simulink model "gm_parallel_8_delay_compensation"  (R2022a)
settings: Solver=FixedStepDiscrete  StartTime=0.0  StopTime=10.0  RelTol=1e-3
undefined symbols (not defined in the file or in its folder): f_c, L_d, L_q, L_x, L_y, p, psi_pm, R_ph
libraries: hdlmdlgenlib x30
settings Model: Creator=Andre Merx  LastModifiedBy=Andre Merx
settings SolverCC: AlgebraicLoopSolver=TrustRegion
settings DataIOCC: LimitDataPoints=on  SaveOutput=off  SaveTime=off
settings OptimizationCC: BlockReduction=off  ConditionallyExecuteInputs=off  DefaultParameterBehavior=Inlined  LifeSpan=inf
settings DebuggingCC: AlgebraicLoopMsg=error  InheritedTsInSrcMsg=none  SingleTaskRateTransMsg=error  UnconnectedInputMsg=warning  UnconnectedOutputMsg=warning  UnconnectedLineMsg=warning  AllowSymbolicDim=off  StrictBusMsg=ErrorOnBusTreatedAsVector  SFUnexpectedBacktrackingDiag=warning  SFNoUnconditionalDefaultTransitionDiag=warning  SFExecutionAtInitializationDiag=none  SFMachineParentedDataDiag=warning  ArithmeticOperatorsInVariantConditions=warning
settings HardwareCC: ProdBitPerPointer=32  ProdBitPerSizeT=32  ProdBitPerPtrDiffT=32  ProdLargestAtomicFloat=None  ProdIntDivRoundTo=Undefined  ProdEndianess=Unspecified  ProdWordSize=32  ProdHWDeviceType=ASIC/FPGA->ASIC/FPGA  ProdEqTarget=off
settings SFSimCC: SimUseLocalCustomCode=off  CustomCodeUndefinedFunction=UseInterfaceOnly
settings RTWCC: RTWUseLocalCustomCode=off
settings CodeAppCC: StateflowObjectComments=on
settings GRTTargetCC: TargetLangStandard=C89/C90 (ANSI)
settings ConfigComp: CovScope=ReferencedModels  CovMetricSettings=dw  CovSaveCumulativeToWorkspaceVar=on  CovSaveSingleToWorkspaceVar=on  CovExternalEMLEnable=off  CovSFcnEnable=off

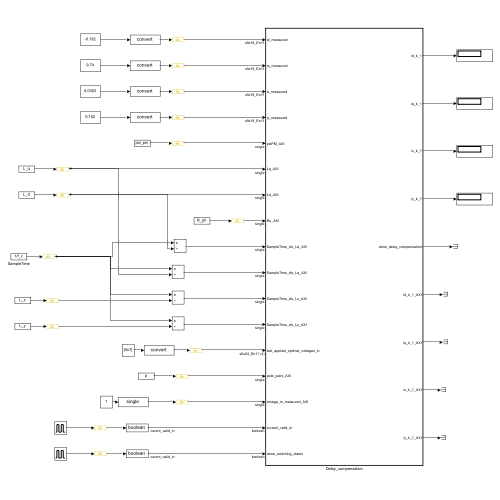
[thumbnail: Simulink's stored preview of the top-level diagram]
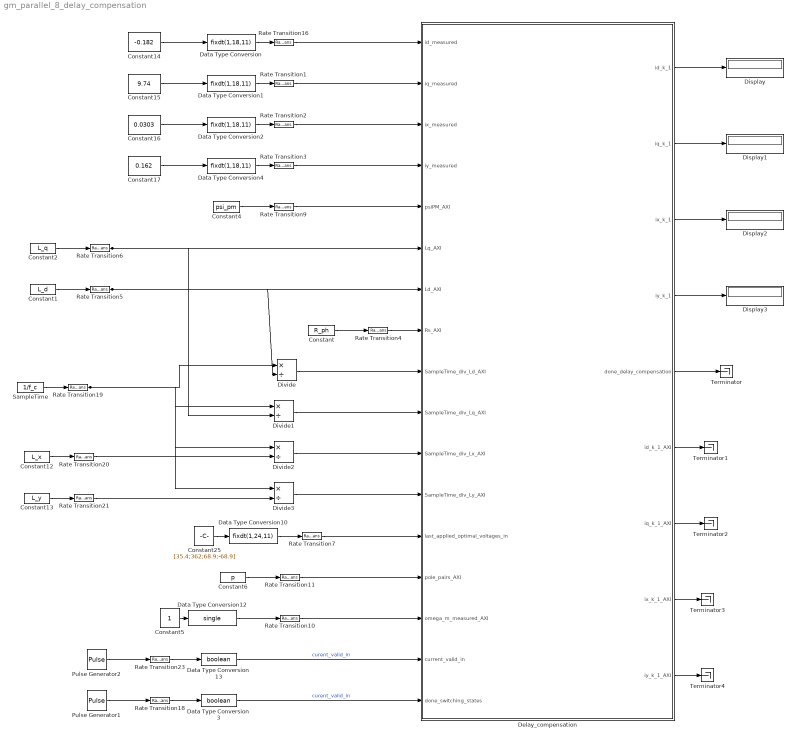
== system gm_parallel_8_delay_compensation ==
  Constant : Constant  Value=R_ph  OutDataTypeStr=single  SampleTime=-1
  Constant1 : Constant  Value=L_d  OutDataTypeStr=single  SampleTime=-1
  Constant12 : Constant  Value=L_x  OutDataTypeStr=single  SampleTime=-1
  Constant13 : Constant  Value=L_y  OutDataTypeStr=single  SampleTime=-1
  Constant14 : Constant  Value=-0.182
  Constant15 : Constant  Value=9.74
  Constant16 : Constant  Value=0.0303
  Constant17 : Constant  Value=0.162
  Constant2 : Constant  Value=L_q  OutDataTypeStr=single  SampleTime=-1
  Constant25 : Constant  Value=[35.4;362;68.9;-68.9]
  Constant4 : Constant  Value=psi_pm  OutDataTypeStr=single  SampleTime=-1
  Constant5 : Constant
  Constant6 : Constant  Value=p  OutDataTypeStr=single  SampleTime=-1
  Data Type Conversion{,1..2,4} (4 alike) : DataTypeConversion  OutDataTypeStr=fixdt(1,18,11)  SaturateOnIntegerOverflow=off  RndMeth=Floor
  Data Type Conversion10 : DataTypeConversion  OutDataTypeStr=fixdt(1,24,11)  SaturateOnIntegerOverflow=off  RndMeth=Floor
  Data Type Conversion12 : DataTypeConversion  OutDataTypeStr=single  SaturateOnIntegerOverflow=off  RndMeth=Floor
  Data Type Conversion13 : DataTypeConversion  OutDataTypeStr=boolean  SaturateOnIntegerOverflow=off  RndMeth=Floor
  Data Type Conversion3 : DataTypeConversion  OutDataTypeStr=boolean  SaturateOnIntegerOverflow=off  RndMeth=Floor
  Delay_compensation : Subsystem  TreatAsAtomicUnit=on
  Display{,1..3} (4 alike) : Display
  Divide{,1..3} (4 alike) : Product  Inputs=*/  RndMeth=Zero  SaturateOnIntegerOverflow=on
  Pulse Generator1 : DiscretePulseGenerator  PulseType=Time based  Period=1/f_c
  Pulse Generator2 : DiscretePulseGenerator  PulseType=Time based  Period=1/f_c
  Rate Transition{1..7,9..11,16,18..21,23} (16 alike) : RateTransition  OutPortSampleTime=Rt
  SampleTime : Constant  Value=1/f_c  OutDataTypeStr=single  SampleTime=-1
  Terminator{,1..4} (5 alike) : Terminator
  wires:
  Delay_compensation/9(iy_k_1_AXI) -> Terminator4/1
  Delay_compensation/8(ix_k_1_AXI) -> Terminator3/1
  Delay_compensation/7(iq_k_1_AXI) -> Terminator2/1
  Delay_compensation/6(id_k_1_AXI) -> Terminator1/1
  Rate Transition6/1 -> Divide1/2, Delay_compensation/6(Lq_AXI)
  Rate Transition9/1 -> Delay_compensation/5(psiPM_AXI)
  Constant2/1 -> Rate Transition6/1
  Divide1/1 -> Delay_compensation/10(SampleTime_div_Lq_AXI)
  Constant14/1 -> Data Type Conversion/1
  Divide/1 -> Delay_compensation/9(SampleTime_div_Ld_AXI)
  Rate Transition20/1 -> Divide2/2
  Constant25/1 -> Data Type Conversion10/1
  Rate Transition11/1 -> Delay_compensation/14(pole_pairs_AXI)
  Rate Transition7/1 -> Delay_compensation/13(last_applied_optimal_voltages_in)
  Constant5/1 -> Data Type Conversion12/1
  Divide2/1 -> Delay_compensation/11(SampleTime_div_Lx_AXI)
  Constant/1 -> Rate Transition4/1
  Data Type Conversion13/1 -> Delay_compensation/16(current_valid_in)  "curent_valid_in"
  Data Type Conversion12/1 -> Rate Transition10/1
  Rate Transition21/1 -> Divide3/2
  Rate Transition3/1 -> Delay_compensation/4(iy_measured)
  Rate Transition10/1 -> Delay_compensation/15(omega_m_measured_AXI)
  Divide3/1 -> Delay_compensation/12(SampleTime_div_Ly_AXI)
  Rate Transition18/1 -> Data Type Conversion3/1
  Constant6/1 -> Rate Transition11/1
  Constant12/1 -> Rate Transition20/1
  Data Type Conversion3/1 -> Delay_compensation/17(done_switching_states)  "curent_valid_in"
  Data Type Conversion4/1 -> Rate Transition3/1
  Rate Transition5/1 -> Divide/2, Delay_compensation/7(Ld_AXI)
  Delay_compensation/2(iq_k_1) -> Display1/1
  Data Type Conversion1/1 -> Rate Transition1/1
  Data Type Conversion10/1 -> Rate Transition7/1
  Data Type Conversion/1 -> Rate Transition16/1
  Data Type Conversion2/1 -> Rate Transition2/1
  Constant15/1 -> Data Type Conversion1/1
  Constant4/1 -> Rate Transition9/1
  Constant16/1 -> Data Type Conversion2/1
  Delay_compensation/3(ix_k_1) -> Display2/1
  Rate Transition1/1 -> Delay_compensation/2(iq_measured)
  Rate Transition2/1 -> Delay_compensation/3(ix_measured)
  Rate Transition4/1 -> Delay_compensation/8(Rs_AXI)
  Constant13/1 -> Rate Transition21/1
  SampleTime/1 -> Rate Transition19/1
  Delay_compensation/1(id_k_1) -> Display/1
  Rate Transition16/1 -> Delay_compensation/1(id_measured)
  Delay_compensation/4(iy_k_1) -> Display3/1
  Pulse Generator1/1 -> Rate Transition18/1
  Delay_compensation/5(done_delay_compensation) -> Terminator/1
  Rate Transition19/1 -> Divide2/1, Divide3/1, Divide1/1, Divide/1
  Pulse Generator2/1 -> Rate Transition23/1
  Constant1/1 -> Rate Transition5/1
  Constant17/1 -> Data Type Conversion4/1
  Rate Transition23/1 -> Data Type Conversion13/1

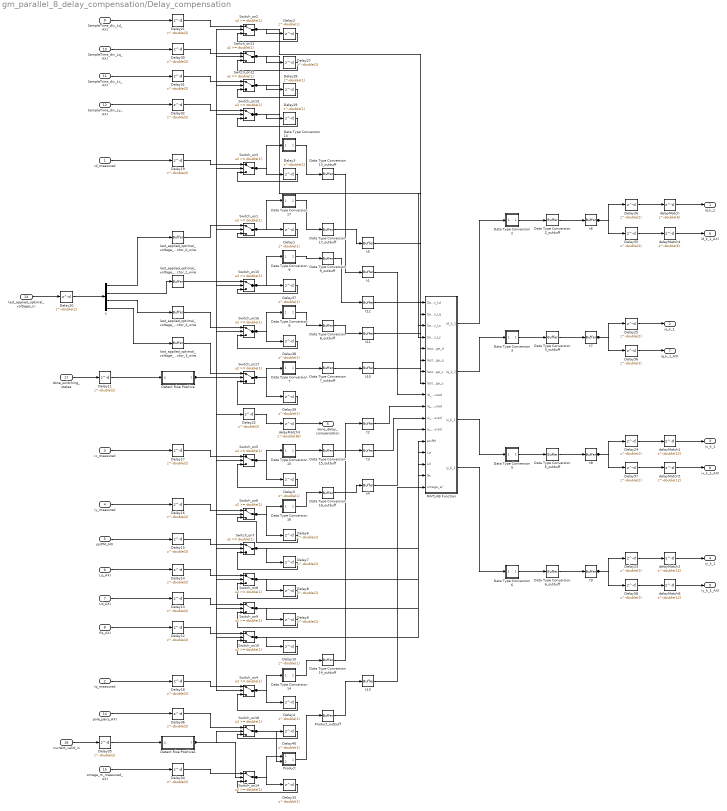
== system gm_parallel_8_delay_compensation/Delay_compensation ==
  id_measured : Inport  OutDataTypeStr=fixdt(1, 18, 11)  PortDimensions=1  SampleTime=1e-08
  iq_measured : Inport  Port=2  OutDataTypeStr=fixdt(1, 18, 11)  PortDimensions=1  SampleTime=1e-08
  ix_measured : Inport  Port=3  OutDataTypeStr=fixdt(1, 18, 11)  PortDimensions=1  SampleTime=1e-08
  iy_measured : Inport  Port=4  OutDataTypeStr=fixdt(1, 18, 11)  PortDimensions=1  SampleTime=1e-08
  psiPM_AXI : Inport  Port=5  OutDataTypeStr=single  PortDimensions=1  SampleTime=1e-08
  Lq_AXI : Inport  Port=6  OutDataTypeStr=single  PortDimensions=1  SampleTime=1e-08
  Ld_AXI : Inport  Port=7  OutDataTypeStr=single  PortDimensions=1  SampleTime=1e-08
  Rs_AXI : Inport  Port=8  OutDataTypeStr=single  PortDimensions=1  SampleTime=1e-08
  SampleTime_div_Ld_AXI : Inport  Port=9  OutDataTypeStr=single  PortDimensions=1  SampleTime=1e-08
  SampleTime_div_Lq_AXI : Inport  Port=10  OutDataTypeStr=single  PortDimensions=1  SampleTime=1e-08
  SampleTime_div_Lx_AXI : Inport  Port=11  OutDataTypeStr=single  PortDimensions=1  SampleTime=1e-08
  SampleTime_div_Ly_AXI : Inport  Port=12  OutDataTypeStr=single  PortDimensions=1  SampleTime=1e-08
  last_applied_optimal_voltages_in : Inport  Port=13  OutDataTypeStr=fixdt(1, 24, 11)  PortDimensions=[4]  SampleTime=1e-08
  pole_pairs_AXI : Inport  Port=14  OutDataTypeStr=single  PortDimensions=1  SampleTime=1e-08
  omega_m_measured_AXI : Inport  Port=15  OutDataTypeStr=single  PortDimensions=1  SampleTime=1e-08
  current_valid_in : Inport  Port=16  OutDataTypeStr=boolean  PortDimensions=1  SampleTime=1e-08
  done_switching_states : Inport  Port=17  OutDataTypeStr=boolean  PortDimensions=1  SampleTime=1e-08
  Data Type Conversion13 : Subsystem
      mask Display: disp('NFP\nconv');
  Data Type Conversion13_outbuff : hdlmdlgenlib/Buffer
      settings: SourceProductBaseCode=SL
  Data Type Conversion14 : Subsystem
      mask Display: disp('NFP\nconv');
  Data Type Conversion14_outbuff : hdlmdlgenlib/Buffer
      settings: SourceProductBaseCode=SL
  Data Type Conversion15 : Subsystem
      mask Display: disp('NFP\nconv');
  Data Type Conversion15_outbuff : hdlmdlgenlib/Buffer
      settings: SourceProductBaseCode=SL
  Data Type Conversion16 : Subsystem
      mask Display: disp('NFP\nconv');
  Data Type Conversion16_outbuff : hdlmdlgenlib/Buffer
      settings: SourceProductBaseCode=SL
  Data Type Conversion17 : Subsystem
      mask Display: disp('NFP\nconv');
  Data Type Conversion17_outbuff : hdlmdlgenlib/Buffer
      settings: SourceProductBaseCode=SL
  Data Type Conversion2 : Subsystem
      mask Display: disp('NFP\nconv');
  Data Type Conversion2_outbuff : hdlmdlgenlib/Buffer
      settings: SourceProductBaseCode=SL
  Data Type Conversion3 : Subsystem
      mask Display: disp('NFP\nconv');
  Data Type Conversion3_outbuff : hdlmdlgenlib/Buffer
      settings: SourceProductBaseCode=SL
  Data Type Conversion5 : Subsystem
      mask Display: disp('NFP\nconv');
  Data Type Conversion5_outbuff : hdlmdlgenlib/Buffer
      settings: SourceProductBaseCode=SL
  Data Type Conversion6 : Subsystem
      mask Display: disp('NFP\nconv');
  Data Type Conversion6_outbuff : hdlmdlgenlib/Buffer
      settings: SourceProductBaseCode=SL
  Data Type Conversion7 : Subsystem
      mask Display: disp('NFP\nconv');
  Data Type Conversion7_outbuff : hdlmdlgenlib/Buffer
      settings: SourceProductBaseCode=SL
  Data Type Conversion8 : Subsystem
      mask Display: disp('NFP\nconv');
  Data Type Conversion8_outbuff : hdlmdlgenlib/Buffer
      settings: SourceProductBaseCode=SL
  Data Type Conversion9 : Subsystem
      mask Display: disp('NFP\nconv');
  Data Type Conversion9_outbuff : hdlmdlgenlib/Buffer
      settings: SourceProductBaseCode=SL
  Delay{1..10,27..29,33,37..40} (18 alike) : Delay  DelayLength=double(1)  InitialCondition=0  SampleTime=1e-08
  Delay{11..26,30..32,34..36,55..58} (26 alike) : Delay  DelayLength=double(2)  InitialCondition=0  SampleTime=1e-08
  Detect Rise Positive : Subsystem  mask(Detect Rise Positive){vinit=double(0), InputProcessing=Elements as channels (sample based), OutDataTypeStr=boolean}
      mask prompts: vinit "Simulink:masks:InitialCondition_MP"; InputProcessing "Simulink:masks:InputProcessing_MP"; OutDataTypeStr "Simulink:masks:OutputDataType_MP"
      mask help: Simulink:masks:DetectRisePositive_MD
      mask init:
      | InputProcessing = 'Elements as channels (sample based)';
      | OutDataTypeStr = 'boolean';
      | vinit = double(0);
      mask TypeOptions InputProcessing: Simulink:masks:ColumnsAsChannelsFrameBased | Simulink:masks:ElementsAsChannelsSampleBased
      mask TypeOptions OutDataTypeStr: Simulink:masks:uint8 | Simulink:masks:boolean
      mask Display: fprintf('U > 0\n&  NOT\nU/z > 0')
  Detect Rise Positive1 : Subsystem  mask(Detect Rise Positive){vinit=double(0), InputProcessing=Elements as channels (sample based), OutDataTypeStr=boolean}
      mask prompts: vinit "Simulink:masks:InitialCondition_MP"; InputProcessing "Simulink:masks:InputProcessing_MP"; OutDataTypeStr "Simulink:masks:OutputDataType_MP"
      mask help: Simulink:masks:DetectRisePositive_MD
      mask init:
      | InputProcessing = 'Elements as channels (sample based)';
      | OutDataTypeStr = 'boolean';
      | vinit = double(0);
      mask TypeOptions InputProcessing: Simulink:masks:ColumnsAsChannelsFrameBased | Simulink:masks:ElementsAsChannelsSampleBased
      mask TypeOptions OutDataTypeStr: Simulink:masks:uint8 | Simulink:masks:boolean
      mask Display: fprintf('U > 0\n&  NOT\nU/z > 0')
  MATLAB Function : Subsystem
  Product : Subsystem
      mask Display: disp('NFP\nmul');
  Product_outbuff : hdlmdlgenlib/Buffer
      settings: SourceProductBaseCode=SL
  Switch_on{1,15..17} (4 alike) : Switch  Threshold=double(1)  OutDataTypeStr=fixdt(1, 24, 11)  RndMeth=Simplest  SampleTime=1e-08  SaturateOnIntegerOverflow=off  InputSameDT=off
  Switch_on{2,7..14,18} (10 alike) : Switch  Threshold=double(1)  OutDataTypeStr=single  RndMeth=Simplest  SampleTime=1e-08  SaturateOnIntegerOverflow=off  InputSameDT=off
  Switch_on{3..6} (4 alike) : Switch  Threshold=double(1)  OutDataTypeStr=fixdt(1, 18, 11)  RndMeth=Simplest  SampleTime=1e-08  SaturateOnIntegerOverflow=off  InputSameDT=off
  delayMatch : Delay  DelayLength=double(6)  InitialCondition=0  SampleTime=1e-08
  delayMatch{1..2,5..6} (4 alike) : Delay  DelayLength=double(12)  InitialCondition=0  SampleTime=1e-08
  delayMatch3 : Delay  DelayLength=double(36)  InitialCondition=0  SampleTime=1e-08
  delayMatch4 : Delay  DelayLength=double(6)  InitialCondition=0  SampleTime=1e-08
  last_applied_optimal_voltage_vector_0_wire : hdlmdlgenlib/Buffer
      settings: SourceProductBaseCode=SL
  last_applied_optimal_voltage_vector_1_wire : hdlmdlgenlib/Buffer
      settings: SourceProductBaseCode=SL
  last_applied_optimal_voltage_vector_2_wire : hdlmdlgenlib/Buffer
      settings: SourceProductBaseCode=SL
  last_applied_optimal_voltage_vector_3_wire : hdlmdlgenlib/Buffer
      settings: SourceProductBaseCode=SL
  t : Demux
  t{1..13} (13 alike) : hdlmdlgenlib/Buffer
      settings: SourceProductBaseCode=SL
  id_k_1 : Outport  SampleTime=1e-08
  iq_k_1 : Outport  Port=2  SampleTime=1e-08
  ix_k_1 : Outport  Port=3  SampleTime=1e-08
  iy_k_1 : Outport  Port=4  SampleTime=1e-08
  done_delay_compensation : Outport  Port=5  SampleTime=1e-08
  id_k_1_AXI : Outport  Port=6  SampleTime=1e-08
  iq_k_1_AXI : Outport  Port=7  SampleTime=1e-08
  ix_k_1_AXI : Outport  Port=8  SampleTime=1e-08
  iy_k_1_AXI : Outport  Port=9  SampleTime=1e-08
  wires:
  id_measured/1 -> Delay19/1
  iq_measured/1 -> Delay18/1
  ix_measured/1 -> Delay17/1
  iy_measured/1 -> Delay16/1
  psiPM_AXI/1 -> Delay15/1
  Lq_AXI/1 -> Delay14/1
  Ld_AXI/1 -> Delay13/1
  Rs_AXI/1 -> Delay12/1
  SampleTime_div_Ld_AXI/1 -> Delay21/1
  SampleTime_div_Lq_AXI/1 -> Delay30/1
  SampleTime_div_Lx_AXI/1 -> Delay31/1
  SampleTime_div_Ly_AXI/1 -> Delay32/1
  last_applied_optimal_voltages_in/1 -> Delay20/1
  pole_pairs_AXI/1 -> Delay36/1
  omega_m_measured_AXI/1 -> Delay34/1
  current_valid_in/1 -> Delay35/1
  done_switching_states/1 -> Delay11/1
  Data Type Conversion13_outbuff/1 -> t1/1
  Data Type Conversion14_outbuff/1 -> t2/1
  Data Type Conversion15_outbuff/1 -> t3/1
  Data Type Conversion16_outbuff/1 -> t4/1
  Data Type Conversion17_outbuff/1 -> t5/1
  Data Type Conversion2_outbuff/1 -> t6/1
  Data Type Conversion3_outbuff/1 -> t7/1
  Data Type Conversion5_outbuff/1 -> t8/1
  Data Type Conversion6_outbuff/1 -> t9/1
  Data Type Conversion7_outbuff/1 -> t10/1
  Data Type Conversion8_outbuff/1 -> t11/1
  Data Type Conversion9_outbuff/1 -> t12/1
  Delay11/1 -> Detect Rise Positive/1(U)
  Delay12/1 -> Switch_on10/1
  Delay13/1 -> Switch_on9/1
  Delay14/1 -> Switch_on8/1
  Delay15/1 -> Switch_on7/1
  Delay16/1 -> Switch_on6/1
  Delay17/1 -> Switch_on5/1
  Delay18/1 -> Switch_on4/1
  Delay19/1 -> Switch_on3/1
  Delay20/1 -> t/1
  Delay21/1 -> Switch_on2/1
  delayMatch3/1 -> done_delay_compensation/1
  delayMatch2/1 -> iy_k_1/1
  delayMatch1/1 -> ix_k_1/1
  Delay25/1 -> iq_k_1/1
  delayMatch/1 -> id_k_1/1
  Delay30/1 -> Switch_on11/1
  Delay31/1 -> Switch_on12/1
  Delay32/1 -> Switch_on13/1
  Delay34/1 -> Switch_on14/1
  Delay35/1 -> Detect Rise Positive1/1(U)
  Delay36/1 -> Switch_on18/1
  t4/1 -> MATLAB Function/12(iy_measured)
  t3/1 -> MATLAB Function/11(ix_measured)
  t2/1 -> MATLAB Function/10(iq_measured)
  t1/1 -> MATLAB Function/9(id_measured)
  t6/1 -> Delay55/1, Delay26/1
  t7/1 -> Delay56/1, Delay25/1
  t8/1 -> Delay57/1, Delay24/1
  t9/1 -> Delay58/1, Delay23/1
  t10/1 -> MATLAB Function/8(last_applied_optimal_voltage_y)
  t11/1 -> MATLAB Function/7(last_applied_optimal_voltage_x)
  t12/1 -> MATLAB Function/6(last_applied_optimal_voltage_q)
  t5/1 -> MATLAB Function/5(last_applied_optimal_voltage_d)
  t13/1 -> MATLAB Function/17(omega_el)
  delayMatch4/1 -> id_k_1_AXI/1
  Delay56/1 -> iq_k_1_AXI/1
  delayMatch5/1 -> ix_k_1_AXI/1
  delayMatch6/1 -> iy_k_1_AXI/1
  last_applied_optimal_voltage_vector_0_wire/1 -> Switch_on1/1
  last_applied_optimal_voltage_vector_1_wire/1 -> Switch_on15/1
  last_applied_optimal_voltage_vector_2_wire/1 -> Switch_on16/1
  last_applied_optimal_voltage_vector_3_wire/1 -> Switch_on17/1
  Detect Rise Positive/1(Y) -> Delay22/1, Switch_on2/2, Switch_on11/2, Switch_on12/2, Switch_on13/2, Switch_on1/2, Switch_on15/2, Switch_on16/2, Switch_on17/2, Switch_on3/2, Switch_on4/2, Switch_on5/2, Switch_on6/2, Switch_on7/2, Switch_on8/2, Switch_on9/2, Switch_on10/2
  Detect Rise Positive1/1(Y) -> Switch_on14/2, Switch_on18/2
  MATLAB Function/1(id_k_1) -> Data Type Conversion2/1(In1)
  MATLAB Function/2(iq_k_1) -> Data Type Conversion3/1(In1)
  MATLAB Function/3(ix_k_1) -> Data Type Conversion5/1(In1)
  MATLAB Function/4(iy_k_1) -> Data Type Conversion6/1(In1)
  Product_outbuff/1 -> t13/1
  Switch_on1/1 -> Data Type Conversion17/1(In1), Delay1/1
  Switch_on10/1 -> MATLAB Function/16(Rs), Delay10/1
  Switch_on11/1 -> MATLAB Function/2(SampleTime_div_Lq), Delay27/1
  Switch_on12/1 -> MATLAB Function/3(SampleTime_div_Lx), Delay28/1
  Switch_on13/1 -> MATLAB Function/4(SampleTime_div_Ly), Delay29/1
  Switch_on14/1 -> Product/1(In1), Delay33/1
  Switch_on15/1 -> Data Type Conversion9/1(In1), Delay37/1
  Switch_on16/1 -> Data Type Conversion8/1(In1), Delay38/1
  Switch_on17/1 -> Data Type Conversion7/1(In1), Delay39/1
  Switch_on18/1 -> Product/2(In2), Delay40/1
  Switch_on2/1 -> MATLAB Function/1(SampleTime_div_Ld), Delay2/1
  Switch_on3/1 -> Data Type Conversion13/1(In1), Delay3/1
  Switch_on4/1 -> Data Type Conversion14/1(In1), Delay4/1
  Switch_on5/1 -> Data Type Conversion15/1(In1), Delay5/1
  Switch_on6/1 -> Data Type Conversion16/1(In1), Delay6/1
  Switch_on7/1 -> MATLAB Function/13(psiPM), Delay7/1
  Switch_on8/1 -> MATLAB Function/14(Lq), Delay8/1
  Switch_on9/1 -> MATLAB Function/15(Ld), Delay9/1
  t/1 -> last_applied_optimal_voltage_vector_0_wire/1
  t/2 -> last_applied_optimal_voltage_vector_1_wire/1
  t/3 -> last_applied_optimal_voltage_vector_2_wire/1
  t/4 -> last_applied_optimal_voltage_vector_3_wire/1
  Delay26/1 -> delayMatch/1
  Delay24/1 -> delayMatch1/1
  Delay23/1 -> delayMatch2/1
  Delay22/1 -> delayMatch3/1
  Delay55/1 -> delayMatch4/1
  Delay57/1 -> delayMatch5/1
  Delay58/1 -> delayMatch6/1
  Data Type Conversion13/1(Out1) -> Data Type Conversion13_outbuff/1
  Data Type Conversion14/1(Out1) -> Data Type Conversion14_outbuff/1
  Data Type Conversion15/1(Out1) -> Data Type Conversion15_outbuff/1
  Data Type Conversion16/1(Out1) -> Data Type Conversion16_outbuff/1
  Data Type Conversion17/1(Out1) -> Data Type Conversion17_outbuff/1
  Data Type Conversion2/1(Out1) -> Data Type Conversion2_outbuff/1
  Data Type Conversion3/1(Out1) -> Data Type Conversion3_outbuff/1
  Data Type Conversion5/1(Out1) -> Data Type Conversion5_outbuff/1
  Data Type Conversion6/1(Out1) -> Data Type Conversion6_outbuff/1
  Data Type Conversion7/1(Out1) -> Data Type Conversion7_outbuff/1
  Data Type Conversion8/1(Out1) -> Data Type Conversion8_outbuff/1
  Data Type Conversion9/1(Out1) -> Data Type Conversion9_outbuff/1
  Product/1(Out1) -> Product_outbuff/1
  Delay2/1 -> Switch_on2/3
  Delay27/1 -> Switch_on11/3
  Delay28/1 -> Switch_on12/3
  Delay29/1 -> Switch_on13/3
  Delay1/1 -> Switch_on1/3
  Delay37/1 -> Switch_on15/3
  Delay38/1 -> Switch_on16/3
  Delay39/1 -> Switch_on17/3
  Delay3/1 -> Switch_on3/3
  Delay4/1 -> Switch_on4/3
  Delay5/1 -> Switch_on5/3
  Delay6/1 -> Switch_on6/3
  Delay7/1 -> Switch_on7/3
  Delay8/1 -> Switch_on8/3
  Delay9/1 -> Switch_on9/3
  Delay10/1 -> Switch_on10/3
  Delay33/1 -> Switch_on14/3
  Delay40/1 -> Switch_on18/3

== system gm_parallel_8_delay_compensation/Delay_compensation/Data Type Conversion13 ==
  In1 : Inport
  Data Type Conversion13 : DataTypeConversion  OutDataTypeStr=single  RndMeth=Nearest  SampleTime=1e-08  SaturateOnIntegerOverflow=off
  Data Type Conversion13_pd1 : Delay  DelayLength=6
  Out1 : Outport
  wires:
  In1/1 -> Data Type Conversion13/1
  Data Type Conversion13/1 -> Data Type Conversion13_pd1/1
  Data Type Conversion13_pd1/1 -> Out1/1

== system gm_parallel_8_delay_compensation/Delay_compensation/Data Type Conversion14 ==
  In1 : Inport
  Data Type Conversion14 : DataTypeConversion  OutDataTypeStr=single  RndMeth=Nearest  SampleTime=1e-08  SaturateOnIntegerOverflow=off
  Data Type Conversion14_pd1 : Delay  DelayLength=6
  Out1 : Outport
  wires:
  In1/1 -> Data Type Conversion14/1
  Data Type Conversion14/1 -> Data Type Conversion14_pd1/1
  Data Type Conversion14_pd1/1 -> Out1/1

== system gm_parallel_8_delay_compensation/Delay_compensation/Data Type Conversion15 ==
  In1 : Inport
  Data Type Conversion15 : DataTypeConversion  OutDataTypeStr=single  RndMeth=Nearest  SampleTime=1e-08  SaturateOnIntegerOverflow=off
  Data Type Conversion15_pd1 : Delay  DelayLength=6
  Out1 : Outport
  wires:
  In1/1 -> Data Type Conversion15/1
  Data Type Conversion15/1 -> Data Type Conversion15_pd1/1
  Data Type Conversion15_pd1/1 -> Out1/1

== system gm_parallel_8_delay_compensation/Delay_compensation/Data Type Conversion16 ==
  In1 : Inport
  Data Type Conversion16 : DataTypeConversion  OutDataTypeStr=single  RndMeth=Nearest  SampleTime=1e-08  SaturateOnIntegerOverflow=off
  Data Type Conversion16_pd1 : Delay  DelayLength=6
  Out1 : Outport
  wires:
  In1/1 -> Data Type Conversion16/1
  Data Type Conversion16/1 -> Data Type Conversion16_pd1/1
  Data Type Conversion16_pd1/1 -> Out1/1

== system gm_parallel_8_delay_compensation/Delay_compensation/Data Type Conversion17 ==
  In1 : Inport
  Data Type Conversion17 : DataTypeConversion  OutDataTypeStr=single  RndMeth=Nearest  SampleTime=1e-08  SaturateOnIntegerOverflow=off
  Data Type Conversion17_pd1 : Delay  DelayLength=6
  Out1 : Outport
  wires:
  In1/1 -> Data Type Conversion17/1
  Data Type Conversion17/1 -> Data Type Conversion17_pd1/1
  Data Type Conversion17_pd1/1 -> Out1/1

== system gm_parallel_8_delay_compensation/Delay_compensation/Data Type Conversion2 ==
  In1 : Inport
  Data Type Conversion2 : DataTypeConversion  OutDataTypeStr=fixdt(1, 18, 11)  SampleTime=1e-08  SaturateOnIntegerOverflow=off  RndMeth=Floor
  Data Type Conversion2_pd1 : Delay  DelayLength=6
  Out1 : Outport
  wires:
  In1/1 -> Data Type Conversion2/1
  Data Type Conversion2/1 -> Data Type Conversion2_pd1/1
  Data Type Conversion2_pd1/1 -> Out1/1

== system gm_parallel_8_delay_compensation/Delay_compensation/Data Type Conversion3 ==
  In1 : Inport
  Data Type Conversion3 : DataTypeConversion  OutDataTypeStr=fixdt(1, 18, 11)  SampleTime=1e-08  SaturateOnIntegerOverflow=off  RndMeth=Floor
  Data Type Conversion3_pd1 : Delay  DelayLength=6
  Out1 : Outport
  wires:
  In1/1 -> Data Type Conversion3/1
  Data Type Conversion3/1 -> Data Type Conversion3_pd1/1
  Data Type Conversion3_pd1/1 -> Out1/1

== system gm_parallel_8_delay_compensation/Delay_compensation/Data Type Conversion5 ==
  In1 : Inport
  Data Type Conversion5 : DataTypeConversion  OutDataTypeStr=fixdt(1, 18, 11)  SampleTime=1e-08  SaturateOnIntegerOverflow=off  RndMeth=Floor
  Data Type Conversion5_pd1 : Delay  DelayLength=6
  Out1 : Outport
  wires:
  In1/1 -> Data Type Conversion5/1
  Data Type Conversion5/1 -> Data Type Conversion5_pd1/1
  Data Type Conversion5_pd1/1 -> Out1/1

== system gm_parallel_8_delay_compensation/Delay_compensation/Data Type Conversion6 ==
  In1 : Inport
  Data Type Conversion6 : DataTypeConversion  OutDataTypeStr=fixdt(1, 18, 11)  SampleTime=1e-08  SaturateOnIntegerOverflow=off  RndMeth=Floor
  Data Type Conversion6_pd1 : Delay  DelayLength=6
  Out1 : Outport
  wires:
  In1/1 -> Data Type Conversion6/1
  Data Type Conversion6/1 -> Data Type Conversion6_pd1/1
  Data Type Conversion6_pd1/1 -> Out1/1

== system gm_parallel_8_delay_compensation/Delay_compensation/Data Type Conversion7 ==
  In1 : Inport
  Data Type Conversion7 : DataTypeConversion  OutDataTypeStr=single  RndMeth=Nearest  SampleTime=1e-08  SaturateOnIntegerOverflow=off
  Data Type Conversion7_pd1 : Delay  DelayLength=6
  Out1 : Outport
  wires:
  In1/1 -> Data Type Conversion7/1
  Data Type Conversion7/1 -> Data Type Conversion7_pd1/1
  Data Type Conversion7_pd1/1 -> Out1/1

== system gm_parallel_8_delay_compensation/Delay_compensation/Data Type Conversion8 ==
  In1 : Inport
  Data Type Conversion8 : DataTypeConversion  OutDataTypeStr=single  RndMeth=Nearest  SampleTime=1e-08  SaturateOnIntegerOverflow=off
  Data Type Conversion8_pd1 : Delay  DelayLength=6
  Out1 : Outport
  wires:
  In1/1 -> Data Type Conversion8/1
  Data Type Conversion8/1 -> Data Type Conversion8_pd1/1
  Data Type Conversion8_pd1/1 -> Out1/1

== system gm_parallel_8_delay_compensation/Delay_compensation/Data Type Conversion9 ==
  In1 : Inport
  Data Type Conversion9 : DataTypeConversion  OutDataTypeStr=single  RndMeth=Nearest  SampleTime=1e-08  SaturateOnIntegerOverflow=off
  Data Type Conversion9_pd1 : Delay  DelayLength=6
  Out1 : Outport
  wires:
  In1/1 -> Data Type Conversion9/1
  Data Type Conversion9/1 -> Data Type Conversion9_pd1/1
  Data Type Conversion9_pd1/1 -> Out1/1

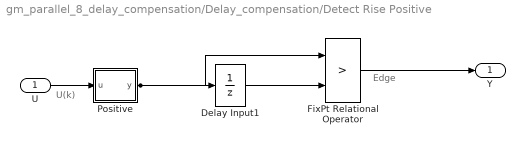
== system gm_parallel_8_delay_compensation/Delay_compensation/Detect Rise Positive ==
  note: Edge
  note: U(k)
  U : Inport  OutDataTypeStr=boolean  SampleTime=1e-08
  Delay Input1 : UnitDelay  Description=Store in Global RAM  DisableCoverage=on  InitialCondition=vinit  SampleTime=-1  HasFrameUpgradeWarning=on
  FixPt Relational Operator : RelationalOperator  Operator=>  OutDataTypeStr=boolean  ZeroCross=off  InputSameDT=off
  Positive : Subsystem  mask(Compare To Zero){relop=>, OutDataTypeStr=boolean, ZeroCross=off}
      mask prompts: relop "Simulink:masks:Operator_MP"; OutDataTypeStr "Simulink:masks:OutputDataType_MP"; ZeroCross "Simulink:masks:EnableZerocrossingDetection_MP"
      mask help: Simulink:masks:CompareToZero_MD
      mask init:
      | OutDataTypeStr = 'boolean';
      | ZeroCross = 'off';
      | blkName = 'parallel_8_delay_compensation/Delay_compensation/Detect Rise\nPositive/Positive';
      | relop = '>';
      | setValue = 'boolean';
      mask TypeOptions relop: == | ~= | < | <= | >= | >
      mask TypeOptions OutDataTypeStr: Simulink:masks:uint8 | Simulink:masks:boolean
      mask Callback ZeroCross: sl('zeroCrossEnable', gcbh);
      mask Display: disp([relop,' 0'])
  Y : Outport  SampleTime=1e-08
  wires:
  Delay Input1/1 -> FixPt Relational Operator/2
  FixPt Relational Operator/1 -> Y/1
  Positive/1(y) -> FixPt Relational Operator/1, Delay Input1/1
  U/1 -> Positive/1(u)

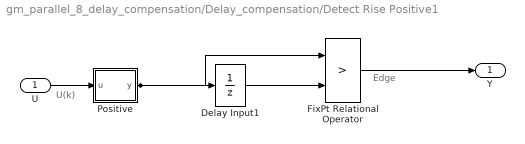
== system gm_parallel_8_delay_compensation/Delay_compensation/Detect Rise Positive1 ==
  note: Edge
  note: U(k)
  U : Inport  OutDataTypeStr=boolean  SampleTime=1e-08
  Delay Input1 : UnitDelay  Description=Store in Global RAM  DisableCoverage=on  InitialCondition=vinit  SampleTime=-1  HasFrameUpgradeWarning=on
  FixPt Relational Operator : RelationalOperator  Operator=>  OutDataTypeStr=boolean  ZeroCross=off  InputSameDT=off
  Positive : Subsystem  mask(Compare To Zero){relop=>, OutDataTypeStr=boolean, ZeroCross=off}
      mask prompts: relop "Simulink:masks:Operator_MP"; OutDataTypeStr "Simulink:masks:OutputDataType_MP"; ZeroCross "Simulink:masks:EnableZerocrossingDetection_MP"
      mask help: Simulink:masks:CompareToZero_MD
      mask init:
      | OutDataTypeStr = 'boolean';
      | ZeroCross = 'off';
      | blkName = 'parallel_8_delay_compensation/Delay_compensation/Detect Rise\nPositive1/Positive';
      | relop = '>';
      | setValue = 'boolean';
      mask TypeOptions relop: == | ~= | < | <= | >= | >
      mask TypeOptions OutDataTypeStr: Simulink:masks:uint8 | Simulink:masks:boolean
      mask Callback ZeroCross: sl('zeroCrossEnable', gcbh);
      mask Display: disp([relop,' 0'])
  Y : Outport  SampleTime=1e-08
  wires:
  Delay Input1/1 -> FixPt Relational Operator/2
  FixPt Relational Operator/1 -> Y/1
  Positive/1(y) -> FixPt Relational Operator/1, Delay Input1/1
  U/1 -> Positive/1(u)

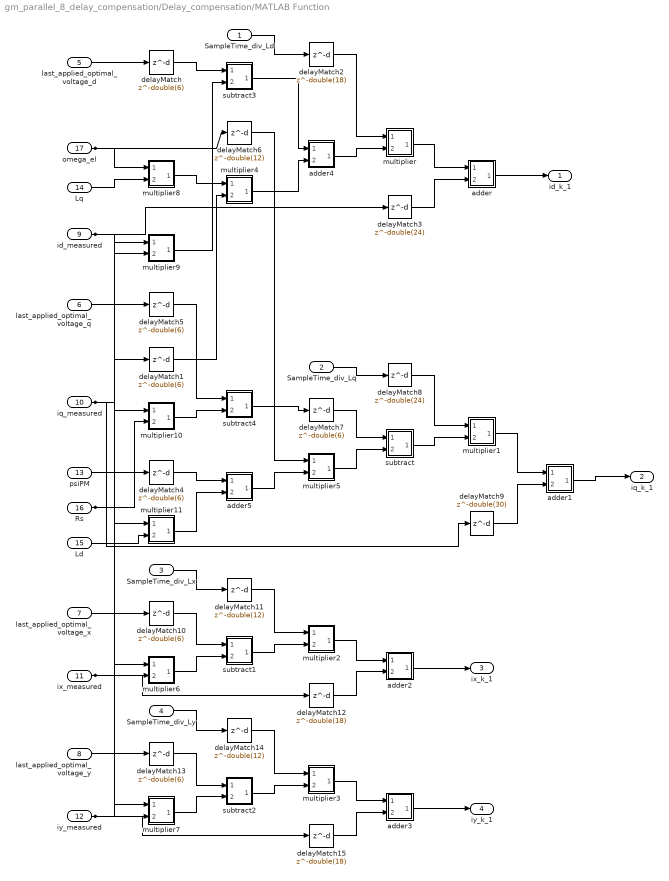
== system gm_parallel_8_delay_compensation/Delay_compensation/MATLAB Function ==
  SampleTime_div_Ld : Inport  OutDataTypeStr=single  PortDimensions=1  SampleTime=1e-08
  SampleTime_div_Lq : Inport  Port=2  OutDataTypeStr=single  PortDimensions=1  SampleTime=1e-08
  SampleTime_div_Lx : Inport  Port=3  OutDataTypeStr=single  PortDimensions=1  SampleTime=1e-08
  SampleTime_div_Ly : Inport  Port=4  OutDataTypeStr=single  PortDimensions=1  SampleTime=1e-08
  last_applied_optimal_voltage_d : Inport  Port=5  OutDataTypeStr=single  PortDimensions=1  SampleTime=1e-08
  last_applied_optimal_voltage_q : Inport  Port=6  OutDataTypeStr=single  PortDimensions=1  SampleTime=1e-08
  last_applied_optimal_voltage_x : Inport  Port=7  OutDataTypeStr=single  PortDimensions=1  SampleTime=1e-08
  last_applied_optimal_voltage_y : Inport  Port=8  OutDataTypeStr=single  PortDimensions=1  SampleTime=1e-08
  id_measured : Inport  Port=9  OutDataTypeStr=single  PortDimensions=1  SampleTime=1e-08
  iq_measured : Inport  Port=10  OutDataTypeStr=single  PortDimensions=1  SampleTime=1e-08
  ix_measured : Inport  Port=11  OutDataTypeStr=single  PortDimensions=1  SampleTime=1e-08
  iy_measured : Inport  Port=12  OutDataTypeStr=single  PortDimensions=1  SampleTime=1e-08
  psiPM : Inport  Port=13  OutDataTypeStr=single  PortDimensions=1  SampleTime=1e-08
  Lq : Inport  Port=14  OutDataTypeStr=single  PortDimensions=1  SampleTime=1e-08
  Ld : Inport  Port=15  OutDataTypeStr=single  PortDimensions=1  SampleTime=1e-08
  Rs : Inport  Port=16  OutDataTypeStr=single  PortDimensions=1  SampleTime=1e-08
  omega_el : Inport  Port=17  OutDataTypeStr=single  PortDimensions=1  SampleTime=1e-08
  adder : Subsystem
      mask Display: disp('NFP\nadd');
  adder1 : Subsystem
      mask Display: disp('NFP\nadd');
  adder2 : Subsystem
      mask Display: disp('NFP\nadd');
  adder3 : Subsystem
      mask Display: disp('NFP\nadd');
  adder4 : Subsystem
      mask Display: disp('NFP\nadd');
  adder5 : Subsystem
      mask Display: disp('NFP\nadd');
  delayMatch{,1,4..5,7,10,13} (7 alike) : Delay  DelayLength=double(6)  InitialCondition=0  SampleTime=1e-08
  delayMatch11 : Delay  DelayLength=double(12)  InitialCondition=0  SampleTime=1e-08
  delayMatch12 : Delay  DelayLength=double(18)  InitialCondition=0  SampleTime=1e-08
  delayMatch14 : Delay  DelayLength=double(12)  InitialCondition=0  SampleTime=1e-08
  delayMatch15 : Delay  DelayLength=double(18)  InitialCondition=0  SampleTime=1e-08
  delayMatch2 : Delay  DelayLength=double(18)  InitialCondition=0  SampleTime=1e-08
  delayMatch3 : Delay  DelayLength=double(24)  InitialCondition=0  SampleTime=1e-08
  delayMatch6 : Delay  DelayLength=double(12)  InitialCondition=0  SampleTime=1e-08
  delayMatch8 : Delay  DelayLength=double(24)  InitialCondition=0  SampleTime=1e-08
  delayMatch9 : Delay  DelayLength=double(30)  InitialCondition=0  SampleTime=1e-08
  multiplier : Subsystem
      mask Display: disp('NFP\nmul');
  multiplier1 : Subsystem
      mask Display: disp('NFP\nmul');
  multiplier10 : Subsystem
      mask Display: disp('NFP\nmul');
  multiplier11 : Subsystem
      mask Display: disp('NFP\nmul');
  multiplier2 : Subsystem
      mask Display: disp('NFP\nmul');
  multiplier3 : Subsystem
      mask Display: disp('NFP\nmul');
  multiplier4 : Subsystem
      mask Display: disp('NFP\nmul');
  multiplier5 : Subsystem
      mask Display: disp('NFP\nmul');
  multiplier6 : Subsystem
      mask Display: disp('NFP\nmul');
  multiplier7 : Subsystem
      mask Display: disp('NFP\nmul');
  multiplier8 : Subsystem
      mask Display: disp('NFP\nmul');
  multiplier9 : Subsystem
      mask Display: disp('NFP\nmul');
  subtract : Subsystem
      mask Display: disp('NFP\nadd');
  subtract1 : Subsystem
      mask Display: disp('NFP\nadd');
  subtract2 : Subsystem
      mask Display: disp('NFP\nadd');
  subtract3 : Subsystem
      mask Display: disp('NFP\nadd');
  subtract4 : Subsystem
      mask Display: disp('NFP\nadd');
  id_k_1 : Outport  SampleTime=1e-08  VectorParamsAs1DForOutWhenUnconnected=off
  iq_k_1 : Outport  Port=2  SampleTime=1e-08
  ix_k_1 : Outport  Port=3  SampleTime=1e-08
  iy_k_1 : Outport  Port=4  SampleTime=1e-08
  wires:
  delayMatch2/1 -> multiplier/1(In1)
  delayMatch8/1 -> multiplier1/1(In1)
  delayMatch11/1 -> multiplier2/1(In1)
  delayMatch14/1 -> multiplier3/1(In1)
  delayMatch/1 -> subtract3/1(In1)
  delayMatch5/1 -> subtract4/1(In1)
  delayMatch10/1 -> subtract1/1(In1)
  delayMatch13/1 -> subtract2/1(In1)
  delayMatch3/1 -> adder/2(In2)
  delayMatch1/1 -> multiplier4/2(In2)
  delayMatch12/1 -> adder2/2(In2)
  delayMatch15/1 -> adder3/2(In2)
  delayMatch4/1 -> adder5/1(In1)
  delayMatch6/1 -> multiplier5/1(In1)
  delayMatch7/1 -> subtract/1(In1)
  adder/1(Out1) -> id_k_1/1
  adder1/1(Out1) -> iq_k_1/1
  adder2/1(Out1) -> ix_k_1/1
  adder3/1(Out1) -> iy_k_1/1
  multiplier/1(Out1) -> adder/1(In1)
  multiplier1/1(Out1) -> adder1/1(In1)
  multiplier2/1(Out1) -> adder2/1(In1)
  multiplier3/1(Out1) -> adder3/1(In1)
  adder4/1(Out1) -> multiplier/2(In2)
  subtract/1(Out1) -> multiplier1/2(In2)
  subtract1/1(Out1) -> multiplier2/2(In2)
  subtract2/1(Out1) -> multiplier3/2(In2)
  multiplier4/1(Out1) -> adder4/2(In2)
  subtract3/1(Out1) -> adder4/1(In1)
  multiplier5/1(Out1) -> subtract/2(In2)
  subtract4/1(Out1) -> delayMatch7/1
  multiplier6/1(Out1) -> subtract1/2(In2)
  multiplier7/1(Out1) -> subtract2/2(In2)
  multiplier8/1(Out1) -> multiplier4/1(In1)
  multiplier9/1(Out1) -> subtract3/2(In2)
  adder5/1(Out1) -> multiplier5/2(In2)
  multiplier10/1(Out1) -> subtract4/2(In2)
  multiplier11/1(Out1) -> adder5/2(In2)
  delayMatch9/1 -> adder1/2(In2)
  SampleTime_div_Ld/1 -> delayMatch2/1
  SampleTime_div_Lq/1 -> delayMatch8/1
  SampleTime_div_Lx/1 -> delayMatch11/1
  SampleTime_div_Ly/1 -> delayMatch14/1
  last_applied_optimal_voltage_d/1 -> delayMatch/1
  last_applied_optimal_voltage_q/1 -> delayMatch5/1
  last_applied_optimal_voltage_x/1 -> delayMatch10/1
  last_applied_optimal_voltage_y/1 -> delayMatch13/1
  id_measured/1 -> delayMatch3/1, multiplier11/1(In1), multiplier9/1(In1)
  iq_measured/1 -> delayMatch9/1, delayMatch1/1, multiplier10/1(In1)
  ix_measured/1 -> delayMatch12/1, multiplier6/1(In1)
  iy_measured/1 -> delayMatch15/1, multiplier7/1(In1)
  psiPM/1 -> delayMatch4/1
  Lq/1 -> multiplier8/2(In2)
  Ld/1 -> multiplier11/2(In2)
  Rs/1 -> multiplier10/2(In2), multiplier9/2(In2), multiplier7/2(In2), multiplier6/2(In2)
  omega_el/1 -> delayMatch6/1, multiplier8/1(In1)

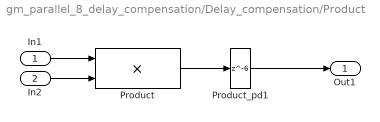
== system gm_parallel_8_delay_compensation/Delay_compensation/Product ==
  In1 : Inport
  In2 : Inport  Port=2
  Product : Product  Inputs=**  OutDataTypeStr=single  SampleTime=1e-08
  Product_pd1 : Delay  DelayLength=6
  Out1 : Outport
  wires:
  In1/1 -> Product/1
  In2/1 -> Product/2
  Product/1 -> Product_pd1/1
  Product_pd1/1 -> Out1/1

== system gm_parallel_8_delay_compensation/Delay_compensation/Detect Rise Positive/Positive ==
  u : Inport  OutDataTypeStr=boolean  SampleTime=1e-08
  Compare : RelationalOperator  Operator=>  OutDataTypeStr=boolean  ZeroCross=off
  Constant : Constant  DisableCoverage=on  Value=0  OutDataTypeStr=Inherit: Inherit via back propagation  SampleTime=-1  PreserveConstantTs=on
  y : Outport  SampleTime=1e-08
  wires:
  Compare/1 -> y/1
  Constant/1 -> Compare/2
  u/1 -> Compare/1

== system gm_parallel_8_delay_compensation/Delay_compensation/Detect Rise Positive1/Positive ==
  u : Inport  OutDataTypeStr=boolean  SampleTime=1e-08
  Compare : RelationalOperator  Operator=>  OutDataTypeStr=boolean  ZeroCross=off
  Constant : Constant  DisableCoverage=on  Value=0  OutDataTypeStr=Inherit: Inherit via back propagation  SampleTime=-1  PreserveConstantTs=on
  y : Outport  SampleTime=1e-08
  wires:
  Compare/1 -> y/1
  Constant/1 -> Compare/2
  u/1 -> Compare/1

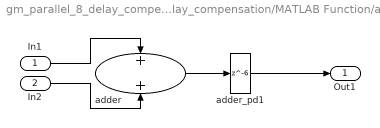
== system gm_parallel_8_delay_compensation/Delay_compensation/MATLAB Function/adder ==
  In1 : Inport
  In2 : Inport  Port=2
  adder : Sum  OutDataTypeStr=single  SampleTime=1e-08
  adder_pd1 : Delay  DelayLength=6
  Out1 : Outport
  wires:
  In1/1 -> adder/1
  In2/1 -> adder/2
  adder/1 -> adder_pd1/1
  adder_pd1/1 -> Out1/1

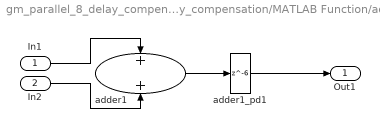
== system gm_parallel_8_delay_compensation/Delay_compensation/MATLAB Function/adder1 ==
  In1 : Inport
  In2 : Inport  Port=2
  adder1 : Sum  OutDataTypeStr=single  SampleTime=1e-08
  adder1_pd1 : Delay  DelayLength=6
  Out1 : Outport
  wires:
  In1/1 -> adder1/1
  In2/1 -> adder1/2
  adder1/1 -> adder1_pd1/1
  adder1_pd1/1 -> Out1/1

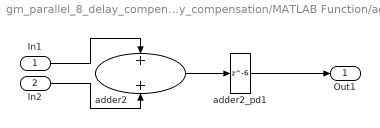
== system gm_parallel_8_delay_compensation/Delay_compensation/MATLAB Function/adder2 ==
  In1 : Inport
  In2 : Inport  Port=2
  adder2 : Sum  OutDataTypeStr=single  SampleTime=1e-08
  adder2_pd1 : Delay  DelayLength=6
  Out1 : Outport
  wires:
  In1/1 -> adder2/1
  In2/1 -> adder2/2
  adder2/1 -> adder2_pd1/1
  adder2_pd1/1 -> Out1/1

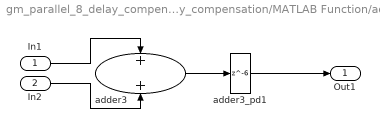
== system gm_parallel_8_delay_compensation/Delay_compensation/MATLAB Function/adder3 ==
  In1 : Inport
  In2 : Inport  Port=2
  adder3 : Sum  OutDataTypeStr=single  SampleTime=1e-08
  adder3_pd1 : Delay  DelayLength=6
  Out1 : Outport
  wires:
  In1/1 -> adder3/1
  In2/1 -> adder3/2
  adder3/1 -> adder3_pd1/1
  adder3_pd1/1 -> Out1/1

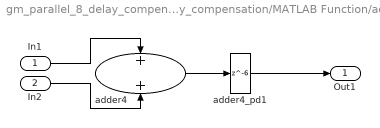
== system gm_parallel_8_delay_compensation/Delay_compensation/MATLAB Function/adder4 ==
  In1 : Inport
  In2 : Inport  Port=2
  adder4 : Sum  OutDataTypeStr=single  SampleTime=1e-08
  adder4_pd1 : Delay  DelayLength=6
  Out1 : Outport
  wires:
  In1/1 -> adder4/1
  In2/1 -> adder4/2
  adder4/1 -> adder4_pd1/1
  adder4_pd1/1 -> Out1/1

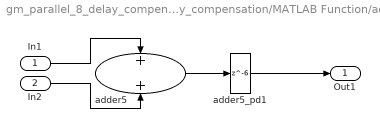
== system gm_parallel_8_delay_compensation/Delay_compensation/MATLAB Function/adder5 ==
  In1 : Inport
  In2 : Inport  Port=2
  adder5 : Sum  OutDataTypeStr=single  SampleTime=1e-08
  adder5_pd1 : Delay  DelayLength=6
  Out1 : Outport
  wires:
  In1/1 -> adder5/1
  In2/1 -> adder5/2
  adder5/1 -> adder5_pd1/1
  adder5_pd1/1 -> Out1/1

== system gm_parallel_8_delay_compensation/Delay_compensation/MATLAB Function/multiplier ==
  In1 : Inport
  In2 : Inport  Port=2
  multiplier : Product  Inputs=**  OutDataTypeStr=single  SampleTime=1e-08
  multiplier_pd1 : Delay  DelayLength=6
  Out1 : Outport
  wires:
  In1/1 -> multiplier/1
  In2/1 -> multiplier/2
  multiplier/1 -> multiplier_pd1/1
  multiplier_pd1/1 -> Out1/1

== system gm_parallel_8_delay_compensation/Delay_compensation/MATLAB Function/multiplier1 ==
  In1 : Inport
  In2 : Inport  Port=2
  multiplier1 : Product  Inputs=**  OutDataTypeStr=single  SampleTime=1e-08
  multiplier1_pd1 : Delay  DelayLength=6
  Out1 : Outport
  wires:
  In1/1 -> multiplier1/1
  In2/1 -> multiplier1/2
  multiplier1/1 -> multiplier1_pd1/1
  multiplier1_pd1/1 -> Out1/1

== system gm_parallel_8_delay_compensation/Delay_compensation/MATLAB Function/multiplier10 ==
  In1 : Inport
  In2 : Inport  Port=2
  multiplier10 : Product  Inputs=**  OutDataTypeStr=single  SampleTime=1e-08
  multiplier10_pd1 : Delay  DelayLength=6
  Out1 : Outport
  wires:
  In1/1 -> multiplier10/1
  In2/1 -> multiplier10/2
  multiplier10/1 -> multiplier10_pd1/1
  multiplier10_pd1/1 -> Out1/1

== system gm_parallel_8_delay_compensation/Delay_compensation/MATLAB Function/multiplier11 ==
  In1 : Inport
  In2 : Inport  Port=2
  multiplier11 : Product  Inputs=**  OutDataTypeStr=single  SampleTime=1e-08
  multiplier11_pd1 : Delay  DelayLength=6
  Out1 : Outport
  wires:
  In1/1 -> multiplier11/1
  In2/1 -> multiplier11/2
  multiplier11/1 -> multiplier11_pd1/1
  multiplier11_pd1/1 -> Out1/1

== system gm_parallel_8_delay_compensation/Delay_compensation/MATLAB Function/multiplier2 ==
  In1 : Inport
  In2 : Inport  Port=2
  multiplier2 : Product  Inputs=**  OutDataTypeStr=single  SampleTime=1e-08
  multiplier2_pd1 : Delay  DelayLength=6
  Out1 : Outport
  wires:
  In1/1 -> multiplier2/1
  In2/1 -> multiplier2/2
  multiplier2/1 -> multiplier2_pd1/1
  multiplier2_pd1/1 -> Out1/1

== system gm_parallel_8_delay_compensation/Delay_compensation/MATLAB Function/multiplier3 ==
  In1 : Inport
  In2 : Inport  Port=2
  multiplier3 : Product  Inputs=**  OutDataTypeStr=single  SampleTime=1e-08
  multiplier3_pd1 : Delay  DelayLength=6
  Out1 : Outport
  wires:
  In1/1 -> multiplier3/1
  In2/1 -> multiplier3/2
  multiplier3/1 -> multiplier3_pd1/1
  multiplier3_pd1/1 -> Out1/1

== system gm_parallel_8_delay_compensation/Delay_compensation/MATLAB Function/multiplier4 ==
  In1 : Inport
  In2 : Inport  Port=2
  multiplier4 : Product  Inputs=**  OutDataTypeStr=single  SampleTime=1e-08
  multiplier4_pd1 : Delay  DelayLength=6
  Out1 : Outport
  wires:
  In1/1 -> multiplier4/1
  In2/1 -> multiplier4/2
  multiplier4/1 -> multiplier4_pd1/1
  multiplier4_pd1/1 -> Out1/1

== system gm_parallel_8_delay_compensation/Delay_compensation/MATLAB Function/multiplier5 ==
  In1 : Inport
  In2 : Inport  Port=2
  multiplier5 : Product  Inputs=**  OutDataTypeStr=single  SampleTime=1e-08
  multiplier5_pd1 : Delay  DelayLength=6
  Out1 : Outport
  wires:
  In1/1 -> multiplier5/1
  In2/1 -> multiplier5/2
  multiplier5/1 -> multiplier5_pd1/1
  multiplier5_pd1/1 -> Out1/1

== system gm_parallel_8_delay_compensation/Delay_compensation/MATLAB Function/multiplier6 ==
  In1 : Inport
  In2 : Inport  Port=2
  multiplier6 : Product  Inputs=**  OutDataTypeStr=single  SampleTime=1e-08
  multiplier6_pd1 : Delay  DelayLength=6
  Out1 : Outport
  wires:
  In1/1 -> multiplier6/1
  In2/1 -> multiplier6/2
  multiplier6/1 -> multiplier6_pd1/1
  multiplier6_pd1/1 -> Out1/1

== system gm_parallel_8_delay_compensation/Delay_compensation/MATLAB Function/multiplier7 ==
  In1 : Inport
  In2 : Inport  Port=2
  multiplier7 : Product  Inputs=**  OutDataTypeStr=single  SampleTime=1e-08
  multiplier7_pd1 : Delay  DelayLength=6
  Out1 : Outport
  wires:
  In1/1 -> multiplier7/1
  In2/1 -> multiplier7/2
  multiplier7/1 -> multiplier7_pd1/1
  multiplier7_pd1/1 -> Out1/1

== system gm_parallel_8_delay_compensation/Delay_compensation/MATLAB Function/multiplier8 ==
  In1 : Inport
  In2 : Inport  Port=2
  multiplier8 : Product  Inputs=**  OutDataTypeStr=single  SampleTime=1e-08
  multiplier8_pd1 : Delay  DelayLength=6
  Out1 : Outport
  wires:
  In1/1 -> multiplier8/1
  In2/1 -> multiplier8/2
  multiplier8/1 -> multiplier8_pd1/1
  multiplier8_pd1/1 -> Out1/1

== system gm_parallel_8_delay_compensation/Delay_compensation/MATLAB Function/multiplier9 ==
  In1 : Inport
  In2 : Inport  Port=2
  multiplier9 : Product  Inputs=**  OutDataTypeStr=single  SampleTime=1e-08
  multiplier9_pd1 : Delay  DelayLength=6
  Out1 : Outport
  wires:
  In1/1 -> multiplier9/1
  In2/1 -> multiplier9/2
  multiplier9/1 -> multiplier9_pd1/1
  multiplier9_pd1/1 -> Out1/1

== system gm_parallel_8_delay_compensation/Delay_compensation/MATLAB Function/subtract ==
  In1 : Inport
  In2 : Inport  Port=2
  subtract : Sum  Inputs=+-  OutDataTypeStr=single  SampleTime=1e-08
  subtract_pd1 : Delay  DelayLength=6
  Out1 : Outport
  wires:
  In1/1 -> subtract/1
  In2/1 -> subtract/2
  subtract/1 -> subtract_pd1/1
  subtract_pd1/1 -> Out1/1

== system gm_parallel_8_delay_compensation/Delay_compensation/MATLAB Function/subtract1 ==
  In1 : Inport
  In2 : Inport  Port=2
  subtract1 : Sum  Inputs=+-  OutDataTypeStr=single  SampleTime=1e-08
  subtract1_pd1 : Delay  DelayLength=6
  Out1 : Outport
  wires:
  In1/1 -> subtract1/1
  In2/1 -> subtract1/2
  subtract1/1 -> subtract1_pd1/1
  subtract1_pd1/1 -> Out1/1

== system gm_parallel_8_delay_compensation/Delay_compensation/MATLAB Function/subtract2 ==
  In1 : Inport
  In2 : Inport  Port=2
  subtract2 : Sum  Inputs=+-  OutDataTypeStr=single  SampleTime=1e-08
  subtract2_pd1 : Delay  DelayLength=6
  Out1 : Outport
  wires:
  In1/1 -> subtract2/1
  In2/1 -> subtract2/2
  subtract2/1 -> subtract2_pd1/1
  subtract2_pd1/1 -> Out1/1

== system gm_parallel_8_delay_compensation/Delay_compensation/MATLAB Function/subtract3 ==
  In1 : Inport
  In2 : Inport  Port=2
  subtract3 : Sum  Inputs=+-  OutDataTypeStr=single  SampleTime=1e-08
  subtract3_pd1 : Delay  DelayLength=6
  Out1 : Outport
  wires:
  In1/1 -> subtract3/1
  In2/1 -> subtract3/2
  subtract3/1 -> subtract3_pd1/1
  subtract3_pd1/1 -> Out1/1

== system gm_parallel_8_delay_compensation/Delay_compensation/MATLAB Function/subtract4 ==
  In1 : Inport
  In2 : Inport  Port=2
  subtract4 : Sum  Inputs=+-  OutDataTypeStr=single  SampleTime=1e-08
  subtract4_pd1 : Delay  DelayLength=6
  Out1 : Outport
  wires:
  In1/1 -> subtract4/1
  In2/1 -> subtract4/2
  subtract4/1 -> subtract4_pd1/1
  subtract4_pd1/1 -> Out1/1
